simulink model "controller"  (R2025a)
settings: Solver=VariableStepAuto  StartTime=0.0  StopTime=20  RelTol=1e-3
values from neighbouring files (symbols this model uses):
  qd = [0 5.20948749525e-05 0.00020837949981 0.000468853874573 0.000833517999241 0.00130237187381 0.00187541549829 0.00255264887267 0.00333407199696 0.00421968487116 0.00520948749525 0.00630347986926 ... (2700 elements, 450x6)]    [dq.mat]
undefined symbols (not defined in the file or in its folder): D, ddqd, dqd, new_time, Q, rou
(part 2 of 2)

== matlab function controller/robot/MATLAB Function2 ==
  data: q input size=6*1; n_hat output size=6*1; dq input size=6*1
function n_hat = fcn(q, dq)
th = q;
dth = dq;
th1 = th(1); th2 = th(2); th3 = th(3); th4 = th(4); th5 = th(5); th6 = th(6);
dth1 = dth(1); dth2 = dth(2); dth3 = dth(3); dth4 = dth(4); dth5 = dth(5); dth6 = dth(6);
% % ddth1 = ddth(1); ddth2 = ddth(2); ddth3 = ddth(3); ddth4 = ddth(4); ddth5 = ddth(5); ddth6 = ddth(6);

G = [0;
    (1866843*sin(th2 - th3 + th4 + th5))/2000000 - (795688119*sin(th2 - th3))/25000000 - (1866843*sin(th2 - th3 + th4 - th5))/2000000 - (40439763*sin(th2 - th3 + th4))/6250000 - (689642019*sin(th2))/12500000;
     (795688119*sin(th2 - th3))/25000000 - (1866843*sin(th2 - th3 + th4 + th5))/2000000 + (1866843*sin(th2 - th3 + th4 - th5))/2000000 + (40439763*sin(th2 - th3 + th4))/6250000;
     (1866843*sin(th2 - th3 + th4 + th5))/2000000 - (1866843*sin(th2 - th3 + th4 - th5))/2000000 - (40439763*sin(th2 - th3 + th4))/6250000;
     (1866843*sin(th2 - th3 + th4 + th5))/2000000 + (1866843*sin(th2 - th3 + th4 - th5))/2000000;
     0];

C = [(138917031*dth2^2*sin(th2))/250000000 - (5709*dth2^2*sin(th2 - th3 + th4 + th5))/2500000 - (5709*dth3^2*sin(th2 - th3 + th4 + th5))/2500000 - (5709*dth4^2*sin(th2 - th3 + th4 + th5))/2500000 - (173173*dth5^2*sin(th2 - th3 + th4 + th5))/5000000 + (2438609*dth2^2*sin(th2 - th3))/6250000 + (2438609*dth3^2*sin(th2 - th3))/6250000 + (378697*dth2^2*sin(th2 - th5))/10000000 - (378697*dth5^2*sin(th2 - th5))/10000000 + (173173*dth2^2*sin(th2 - th3 + th4 - th5))/5000000 + (2389*dth2^2*sin(th2 - th3 + th4 - 2*th5))/1250000 - (2389*dth2^2*sin(th2 - th3 + th4 + 2*th5))/1250000 + (173173*dth3^2*sin(th2 - th3 + th4 - th5))/5000000 + (2389*dth3^2*sin(th2 - th3 + th4 - 2*th5))/1250000 - (2389*dth3^2*sin(th2 - th3 + th4 + 2*th5))/1250000 + (173173*dth4^2*sin(th2 - th3 + th4 - th5))/5000000 + (2389*dth4^2*sin(th2 - th3 + th4 - 2*th5))/1250000 - (2389*dth4^2*sin(th2 - th3 + th4 + 2*th5))/1250000 + (5709*dth5^2*sin(th2 - th3 + th4 - th5))/2500000 + (3998631*dth2^2*sin(th2 - th3 + th4))/31250000 + (17127*dth2^2*sin(th2 - th3 + th5))/500000 - (17127*dth2^2*sin(th3 - th2 + th5))/500000 + (3998631*dth3^2*sin(th2 - th3 + th4))/31250000 + (17127*dth3^2*sin(th2 - th3 + th5))/500000 - (17127*dth3^2*sin(th3 - th2 + th5))/500000 + (3998631*dth4^2*sin(th2 - th3 + th4))/31250000 - (17127*dth5^2*sin(th2 - th3 + th5))/500000 + (17127*dth5^2*sin(th3 - th2 + th5))/500000 + (378697*dth2^2*sin(th2 + th5))/10000000 - (378697*dth5^2*sin(th2 + th5))/10000000 - (161408701*dth1*dth3*sin(th3))/125000000 - (371007*dth1*dth4*sin(th4))/1562500 - (184591*dth1*dth5*sin(th5))/2500000 + (8203377*dth1*dth2*sin(2*th2 - th3 + th4))/15625000 + (371007*dth1*dth2*sin(2*th2 - 2*th3 + th4))/781250 - (8203377*dth1*dth3*sin(2*th2 - th3 + th4))/31250000 - (371007*dth1*dth3*sin(2*th2 - 2*th3 + th4))/781250 + (8203377*dth1*dth4*sin(2*th2 - th3 + th4))/31250000 + (371007*dth1*dth4*sin(2*th2 - 2*th3 + th4))/1562500 + (5709*dth2*dth3*sin(th2 - th3 + th4 + th5))/1250000 - (5709*dth2*dth4*sin(th2 - th3 + th4 + th5))/1250000 - (184591*dth2*dth5*sin(th2 - th3 + th4 + th5))/5000000 + (5709*dth3*dth4*sin(th2 - th3 + th4 + th5))/1250000 + (dth2*dth6*sin(th2 - th3 + th4 + th5))/20000 + (184591*dth3*dth5*sin(th2 - th3 + th4 + th5))/5000000 - (dth3*dth6*sin(th2 - th3 + th4 + th5))/20000 - (184591*dth4*dth5*sin(th2 - th3 + th4 + th5))/5000000 + (dth4*dth6*sin(th2 - th3 + th4 + th5))/20000 + (dth5*dth6*sin(th2 - th3 + th4 + th5))/20000 - (2438609*dth2*dth3*sin(th2 - th3))/3125000 - (8203377*dth1*dth3*sin(th3 - th4))/31250000 + (8203377*dth1*dth4*sin(th3 - th4))/31250000 - (17127*dth1*dth4*sin(th4 - th5))/500000 + (17127*dth1*dth5*sin(th4 - th5))/500000 + (32351*dth1*dth2*sin(2*th2 - 2*th3 + 2*th4 - th5))/1000000 + (2389*dth1*dth2*sin(2*th2 - 2*th3 + 2*th4 - 2*th5))/1250000 + (2389*dth1*dth2*sin(2*th2 - 2*th3 + 2*th4 + 2*th5))/1250000 - (32351*dth1*dth3*sin(2*th2 - 2*th3 + 2*th4 - th5))/1000000 - (2389*dth1*dth3*sin(2*th2 - 2*th3 + 2*th4 - 2*th5))/1250000 - (2389*dth1*dth3*sin(2*th2 - 2*th3 + 2*th4 + 2*th5))/1250000 + (32351*dth1*dth4*sin(2*th2 - 2*th3 + 2*th4 - th5))/1000000 + (2389*dth1*dth4*sin(2*th2 - 2*th3 + 2*th4 - 2*th5))/1250000 + (2389*dth1*dth4*sin(2*th2 - 2*th3 + 2*th4 + 2*th5))/1250000 - (32351*dth1*dth5*sin(2*th2 - 2*th3 + 2*th4 - th5))/2000000 - (2389*dth1*dth5*sin(2*th2 - 2*th3 + 2*th4 - 2*th5))/1250000 + (2389*dth1*dth5*sin(2*th2 - 2*th3 + 2*th4 + 2*th5))/1250000 + (212507419*dth1*dth2*sin(2*th2))/125000000 - (2389*dth1*dth5*sin(2*th5))/625000 + (526847*dth1*dth2*sin(2*th2 - 2*th3 + 2*th4))/6250000 - (526847*dth1*dth3*sin(2*th2 - 2*th3 + 2*th4))/6250000 + (526847*dth1*dth4*sin(2*th2 - 2*th3 + 2*th4))/6250000 - (378697*dth1*dth2*sin(2*th2 - th3 + th4 + th5))/5000000 - (17127*dth1*dth2*sin(2*th2 - 2*th3 + th4 + th5))/250000 + (378697*dth1*dth3*sin(2*th2 - th3 + th4 + th5))/10000000 - (173173*dth2*dth3*sin(th2 - th3 + th4 - th5))/2500000 + (17127*dth1*dth3*sin(2*th2 - 2*th3 + th4 + th5))/250000 - (378697*dth1*dth4*sin(2*th2 - th3 + th4 + th5))/10000000 - (2389*dth2*dth3*sin(th2 - th3 + th4 - 2*th5))/625000 + (2389*dth2*dth3*sin(th2 - th3 + th4 + 2*th5))/625000 + (173173*dth2*dth4*sin(th2 - th3 + th4 - th5))/2500000 - (17127*dth1*dth4*sin(2*th2 - 2*th3 + th4 + th5))/500000 - (378697*dth1*dth5*sin(2*th2 - th3 + th4 + th5))/10000000 + (2389*dth2*dth4*sin(th2 - th3 + th4 - 2*th5))/625000 - (2389*dth2*dth4*sin(th2 - th3 + th4 + 2*th5))/625000 - (184591*dth2*dth5*sin(th2 - th3 + th4 - th5))/5000000 - (173173*dth3*dth4*sin(th2 - th3 + th4 - th5))/2500000 - (17127*dth1*dth5*sin(2*th2 - 2*th3 + th4 + th5))/500000 - (2389*dth2*dth5*sin(th2 - th3 + th4 - 2*th5))/625000 - (2389*dth2*dth5*sin(th2 - th3 + th4 + 2*th5))/625000 - (dth2*dth6*sin(th2 - th3 + th4 - th5))/20000 - (2389*dth3*dth4*sin(th2 - th3 + th4 - 2*th5))/625000 + (2389*dth3*dth4*sin(th2 - th3 + th4 + 2*th5))/625000 + (184591*dth3*dth5*sin(th2 - th3 + th4 - th5))/5000000 + (2389*dth3*dth5*sin(th2 - th3 + th4 - 2*th5))/625000 + (2389*dth3*dth5*sin(th2 - th3 + th4 + 2*th5))/625000 + (dth3*dth6*sin(th2 - th3 + th4 - th5))/20000 - (184591*dth4*dth5*sin(th2 - th3 + th4 - th5))/5000000 - (2389*dth4*dth5*sin(th2 - th3 + th4 - 2*th5))/625000 - (2389*dth4*dth5*sin(th2 - th3 + th4 + 2*th5))/625000 - (dth4*dth6*sin(th2 - th3 + th4 - th5))/20000 + (dth5*dth6*sin(th2 - th3 + th4 - th5))/20000 + (161408701*dth1*dth2*sin(2*th2 - th3))/62500000 + (509639*dth1*dth2*sin(2*th2 - 2*th3))/625000 - (161408701*dth1*dth3*sin(2*th2 - th3))/125000000 - (509639*dth1*dth3*sin(2*th2 - 2*th3))/625000 - (3998631*dth2*dth3*sin(th2 - th3 + th4))/15625000 - (17127*dth2*dth3*sin(th2 - th3 + th5))/250000 + (17127*dth2*dth3*sin(th3 - th2 + th5))/250000 + (3998631*dth2*dth4*sin(th2 - th3 + th4))/15625000 - (378697*dth1*dth3*sin(th3 - th4 + th5))/10000000 - (378697*dth1*dth3*sin(th4 - th3 + th5))/10000000 - (13431*dth2*dth5*sin(th2 - th3 + th4))/1250000 - (3998631*dth3*dth4*sin(th2 - th3 + th4))/15625000 + (378697*dth1*dth4*sin(th3 - th4 + th5))/10000000 + (378697*dth1*dth4*sin(th4 - th3 + th5))/10000000 + (13431*dth3*dth5*sin(th2 - th3 + th4))/1250000 - (378697*dth1*dth5*sin(th3 - th4 + th5))/10000000 + (378697*dth1*dth5*sin(th4 - th3 + th5))/10000000 - (13431*dth4*dth5*sin(th2 - th3 + th4))/1250000 + (17127*dth1*dth4*sin(th4 + th5))/500000 + (17127*dth1*dth5*sin(th4 + th5))/500000 + (378697*dth1*dth2*sin(2*th2 - th3 + th4 - th5))/5000000 + (17127*dth1*dth2*sin(2*th2 - 2*th3 + th4 - th5))/250000 - (378697*dth1*dth3*sin(2*th2 - th3 + th4 - th5))/10000000 - (32351*dth1*dth2*sin(2*th2 - 2*th3 + 2*th4 + th5))/1000000 - (17127*dth1*dth3*sin(2*th2 - 2*th3 + th4 - th5))/250000 + (378697*dth1*dth4*sin(2*th2 - th3 + th4 - th5))/10000000 + (32351*dth1*dth3*sin(2*th2 - 2*th3 + 2*th4 + th5))/1000000 + (17127*dth1*dth4*sin(2*th2 - 2*th3 + th4 - th5))/500000 - (378697*dth1*dth5*sin(2*th2 - th3 + th4 - th5))/10000000 - (32351*dth1*dth4*sin(2*th2 - 2*th3 + 2*th4 + th5))/1000000 - (17127*dth1*dth5*sin(2*th2 - 2*th3 + th4 - th5))/500000 - (32351*dth1*dth5*sin(2*th2 - 2*th3 + 2*th4 + th5))/2000000;
(161408701*dth3^2*sin(th3))/125000000 - (371007*dth4^2*sin(th4))/1562500 + (32351*dth5^2*sin(th5))/1000000 - (8203377*dth1^2*sin(2*th2 - th3 + th4))/31250000 - (371007*dth1^2*sin(2*th2 - 2*th3 + th4))/1562500 + (8203377*dth3^2*sin(th3 - th4))/31250000 + (8203377*dth4^2*sin(th3 - th4))/31250000 - (17127*dth4^2*sin(th4 - th5))/500000 - (17127*dth5^2*sin(th4 - th5))/500000 - (32351*dth1^2*sin(2*th2 - 2*th3 + 2*th4 - th5))/2000000 - (2389*dth1^2*sin(2*th2 - 2*th3 + 2*th4 - 2*th5))/2500000 - (2389*dth1^2*sin(2*th2 - 2*th3 + 2*th4 + 2*th5))/2500000 - (212507419*dth1^2*sin(2*th2))/250000000 - (526847*dth1^2*sin(2*th2 - 2*th3 + 2*th4))/12500000 + (378697*dth1^2*sin(2*th2 - th3 + th4 + th5))/10000000 + (17127*dth1^2*sin(2*th2 - 2*th3 + th4 + th5))/500000 - (161408701*dth1^2*sin(2*th2 - th3))/125000000 - (509639*dth1^2*sin(2*th2 - 2*th3))/1250000 + (378697*dth3^2*sin(th3 - th4 + th5))/10000000 + (378697*dth3^2*sin(th4 - th3 + th5))/10000000 + (378697*dth4^2*sin(th3 - th4 + th5))/10000000 + (378697*dth4^2*sin(th4 - th3 + th5))/10000000 + (378697*dth5^2*sin(th3 - th4 + th5))/10000000 + (378697*dth5^2*sin(th4 - th3 + th5))/10000000 + (17127*dth4^2*sin(th4 + th5))/500000 + (17127*dth5^2*sin(th4 + th5))/500000 - (378697*dth1^2*sin(2*th2 - th3 + th4 - th5))/10000000 - (17127*dth1^2*sin(2*th2 - 2*th3 + th4 - th5))/500000 + (32351*dth1^2*sin(2*th2 - 2*th3 + 2*th4 + th5))/2000000 - (161408701*dth2*dth3*sin(th3))/62500000 - (371007*dth2*dth4*sin(th4))/781250 + (371007*dth3*dth4*sin(th4))/781250 - (dth5*dth6*sin(th5))/10000 + (32351*dth1*dth5*sin(th2 - th3 + th4 + th5))/1000000 - (dth1*dth6*sin(th2 - th3 + th4 + th5))/20000 - (8203377*dth2*dth3*sin(th3 - th4))/15625000 - (378697*dth1*dth5*sin(th2 - th5))/5000000 + (8203377*dth2*dth4*sin(th3 - th4))/15625000 - (8203377*dth3*dth4*sin(th3 - th4))/15625000 - (17127*dth2*dth4*sin(th4 - th5))/250000 + (17127*dth2*dth5*sin(th4 - th5))/250000 + (17127*dth3*dth4*sin(th4 - th5))/250000 - (17127*dth3*dth5*sin(th4 - th5))/250000 + (17127*dth4*dth5*sin(th4 - th5))/250000 + (2389*dth2*dth5*sin(2*th5))/312500 - (2389*dth3*dth5*sin(2*th5))/312500 + (2389*dth4*dth5*sin(2*th5))/312500 - (32351*dth1*dth5*sin(th2 - th3 + th4 - th5))/1000000 - (2389*dth1*dth5*sin(th2 - th3 + th4 - 2*th5))/625000 - (2389*dth1*dth5*sin(th2 - th3 + th4 + 2*th5))/625000 + (dth1*dth6*sin(th2 - th3 + th4 - th5))/20000 + (13431*dth1*dth5*sin(th2 - th3 + th4))/1250000 + (17127*dth1*dth5*sin(th2 - th3 + th5))/250000 + (17127*dth1*dth5*sin(th3 - th2 + th5))/250000 - (378697*dth2*dth3*sin(th3 - th4 + th5))/5000000 - (378697*dth2*dth3*sin(th4 - th3 + th5))/5000000 + (378697*dth2*dth4*sin(th3 - th4 + th5))/5000000 + (378697*dth2*dth4*sin(th4 - th3 + th5))/5000000 - (378697*dth2*dth5*sin(th3 - th4 + th5))/5000000 + (378697*dth2*dth5*sin(th4 - th3 + th5))/5000000 - (378697*dth3*dth4*sin(th3 - th4 + th5))/5000000 - (378697*dth3*dth4*sin(th4 - th3 + th5))/5000000 + (378697*dth3*dth5*sin(th3 - th4 + th5))/5000000 - (378697*dth3*dth5*sin(th4 - th3 + th5))/5000000 - (378697*dth4*dth5*sin(th3 - th4 + th5))/5000000 + (378697*dth4*dth5*sin(th4 - th3 + th5))/5000000 + (378697*dth1*dth5*sin(th2 + th5))/5000000 + (17127*dth2*dth4*sin(th4 + th5))/250000 + (17127*dth2*dth5*sin(th4 + th5))/250000 - (17127*dth3*dth4*sin(th4 + th5))/250000 - (17127*dth3*dth5*sin(th4 + th5))/250000 + (17127*dth4*dth5*sin(th4 + th5))/250000;
(161408701*dth1^2*sin(th3))/250000000 + (161408701*dth2^2*sin(th3))/125000000 + (371007*dth4^2*sin(th4))/1562500 - (32351*dth5^2*sin(th5))/1000000 + (8203377*dth1^2*sin(2*th2 - th3 + th4))/62500000 + (371007*dth1^2*sin(2*th2 - 2*th3 + th4))/1562500 + (8203377*dth1^2*sin(th3 - th4))/62500000 + (8203377*dth2^2*sin(th3 - th4))/31250000 + (17127*dth4^2*sin(th4 - th5))/500000 + (17127*dth5^2*sin(th4 - th5))/500000 + (32351*dth1^2*sin(2*th2 - 2*th3 + 2*th4 - th5))/2000000 + (2389*dth1^2*sin(2*th2 - 2*th3 + 2*th4 - 2*th5))/2500000 + (2389*dth1^2*sin(2*th2 - 2*th3 + 2*th4 + 2*th5))/2500000 + (526847*dth1^2*sin(2*th2 - 2*th3 + 2*th4))/12500000 - (378697*dth1^2*sin(2*th2 - th3 + th4 + th5))/20000000 - (17127*dth1^2*sin(2*th2 - 2*th3 + th4 + th5))/500000 + (161408701*dth1^2*sin(2*th2 - th3))/250000000 + (509639*dth1^2*sin(2*th2 - 2*th3))/1250000 + (378697*dth1^2*sin(th3 - th4 + th5))/20000000 + (378697*dth1^2*sin(th4 - th3 + th5))/20000000 + (378697*dth2^2*sin(th3 - th4 + th5))/10000000 + (378697*dth2^2*sin(th4 - th3 + th5))/10000000 - (17127*dth4^2*sin(th4 + th5))/500000 - (17127*dth5^2*sin(th4 + th5))/500000 + (378697*dth1^2*sin(2*th2 - th3 + th4 - th5))/20000000 + (17127*dth1^2*sin(2*th2 - 2*th3 + th4 - th5))/500000 - (32351*dth1^2*sin(2*th2 - 2*th3 + 2*th4 + th5))/2000000 + (371007*dth2*dth4*sin(th4))/781250 - (371007*dth3*dth4*sin(th4))/781250 + (dth5*dth6*sin(th5))/10000 - (32351*dth1*dth5*sin(th2 - th3 + th4 + th5))/1000000 + (dth1*dth6*sin(th2 - th3 + th4 + th5))/20000 + (17127*dth2*dth4*sin(th4 - th5))/250000 - (17127*dth2*dth5*sin(th4 - th5))/250000 - (17127*dth3*dth4*sin(th4 - th5))/250000 + (17127*dth3*dth5*sin(th4 - th5))/250000 - (17127*dth4*dth5*sin(th4 - th5))/250000 - (2389*dth2*dth5*sin(2*th5))/312500 + (2389*dth3*dth5*sin(2*th5))/312500 - (2389*dth4*dth5*sin(2*th5))/312500 + (32351*dth1*dth5*sin(th2 - th3 + th4 - th5))/1000000 + (2389*dth1*dth5*sin(th2 - th3 + th4 - 2*th5))/625000 + (2389*dth1*dth5*sin(th2 - th3 + th4 + 2*th5))/625000 - (dth1*dth6*sin(th2 - th3 + th4 - th5))/20000 - (13431*dth1*dth5*sin(th2 - th3 + th4))/1250000 - (17127*dth1*dth5*sin(th2 - th3 + th5))/250000 - (17127*dth1*dth5*sin(th3 - th2 + th5))/250000 - (17127*dth2*dth4*sin(th4 + th5))/250000 - (17127*dth2*dth5*sin(th4 + th5))/250000 + (17127*dth3*dth4*sin(th4 + th5))/250000 + (17127*dth3*dth5*sin(th4 + th5))/250000 - (17127*dth4*dth5*sin(th4 + th5))/250000;
(371007*dth1^2*sin(th4))/3125000 + (371007*dth2^2*sin(th4))/1562500 + (371007*dth3^2*sin(th4))/1562500 + (32351*dth5^2*sin(th5))/1000000 - (8203377*dth1^2*sin(2*th2 - th3 + th4))/62500000 - (371007*dth1^2*sin(2*th2 - 2*th3 + th4))/3125000 - (8203377*dth1^2*sin(th3 - th4))/62500000 - (8203377*dth2^2*sin(th3 - th4))/31250000 + (17127*dth1^2*sin(th4 - th5))/1000000 + (17127*dth2^2*sin(th4 - th5))/500000 + (17127*dth3^2*sin(th4 - th5))/500000 - (32351*dth1^2*sin(2*th2 - 2*th3 + 2*th4 - th5))/2000000 - (2389*dth1^2*sin(2*th2 - 2*th3 + 2*th4 - 2*th5))/2500000 - (2389*dth1^2*sin(2*th2 - 2*th3 + 2*th4 + 2*th5))/2500000 - (526847*dth1^2*sin(2*th2 - 2*th3 + 2*th4))/12500000 + (378697*dth1^2*sin(2*th2 - th3 + th4 + th5))/20000000 + (17127*dth1^2*sin(2*th2 - 2*th3 + th4 + th5))/1000000 - (378697*dth1^2*sin(th3 - th4 + th5))/20000000 - (378697*dth1^2*sin(th4 - th3 + th5))/20000000 - (378697*dth2^2*sin(th3 - th4 + th5))/10000000 - (378697*dth2^2*sin(th4 - th3 + th5))/10000000 - (17127*dth1^2*sin(th4 + th5))/1000000 - (17127*dth2^2*sin(th4 + th5))/500000 - (17127*dth3^2*sin(th4 + th5))/500000 - (378697*dth1^2*sin(2*th2 - th3 + th4 - th5))/20000000 - (17127*dth1^2*sin(2*th2 - 2*th3 + th4 - th5))/1000000 + (32351*dth1^2*sin(2*th2 - 2*th3 + 2*th4 + th5))/2000000 - (371007*dth2*dth3*sin(th4))/781250 - (dth5*dth6*sin(th5))/10000 + (32351*dth1*dth5*sin(th2 - th3 + th4 + th5))/1000000 - (dth1*dth6*sin(th2 - th3 + th4 + th5))/20000 - (17127*dth2*dth3*sin(th4 - th5))/250000 + (2389*dth2*dth5*sin(2*th5))/312500 - (2389*dth3*dth5*sin(2*th5))/312500 + (2389*dth4*dth5*sin(2*th5))/312500 - (32351*dth1*dth5*sin(th2 - th3 + th4 - th5))/1000000 - (2389*dth1*dth5*sin(th2 - th3 + th4 - 2*th5))/625000 - (2389*dth1*dth5*sin(th2 - th3 + th4 + 2*th5))/625000 + (dth1*dth6*sin(th2 - th3 + th4 - th5))/20000 + (13431*dth1*dth5*sin(th2 - th3 + th4))/1250000 + (17127*dth2*dth3*sin(th4 + th5))/250000;
(184591*dth1^2*sin(th5))/5000000 - (17127*dth1^2*sin(th4 - th5))/1000000 - (17127*dth2^2*sin(th4 - th5))/500000 - (17127*dth3^2*sin(th4 - th5))/500000 + (32351*dth1^2*sin(2*th2 - 2*th3 + 2*th4 - th5))/4000000 + (2389*dth1^2*sin(2*th2 - 2*th3 + 2*th4 - 2*th5))/2500000 - (2389*dth1^2*sin(2*th2 - 2*th3 + 2*th4 + 2*th5))/2500000 + (2389*dth1^2*sin(2*th5))/1250000 - (2389*dth2^2*sin(2*th5))/625000 - (2389*dth3^2*sin(2*th5))/625000 - (2389*dth4^2*sin(2*th5))/625000 + (378697*dth1^2*sin(2*th2 - th3 + th4 + th5))/20000000 + (17127*dth1^2*sin(2*th2 - 2*th3 + th4 + th5))/1000000 + (378697*dth1^2*sin(th3 - th4 + th5))/20000000 - (378697*dth1^2*sin(th4 - th3 + th5))/20000000 + (378697*dth2^2*sin(th3 - th4 + th5))/10000000 - (378697*dth2^2*sin(th4 - th3 + th5))/10000000 - (17127*dth1^2*sin(th4 + th5))/1000000 - (17127*dth2^2*sin(th4 + th5))/500000 - (17127*dth3^2*sin(th4 + th5))/500000 + (378697*dth1^2*sin(2*th2 - th3 + th4 - th5))/20000000 + (17127*dth1^2*sin(2*th2 - 2*th3 + th4 - th5))/1000000 + (32351*dth1^2*sin(2*th2 - 2*th3 + 2*th4 + th5))/4000000 + (dth2*dth6*sin(th5))/10000 - (dth3*dth6*sin(th5))/10000 + (dth4*dth6*sin(th5))/10000 - (32351*dth1*dth2*sin(th2 - th3 + th4 + th5))/1000000 + (32351*dth1*dth3*sin(th2 - th3 + th4 + th5))/1000000 - (32351*dth1*dth4*sin(th2 - th3 + th4 + th5))/1000000 - (dth1*dth6*sin(th2 - th3 + th4 + th5))/20000 + (378697*dth1*dth2*sin(th2 - th5))/5000000 + (17127*dth2*dth3*sin(th4 - th5))/250000 + (2389*dth2*dth3*sin(2*th5))/312500 - (2389*dth2*dth4*sin(2*th5))/312500 + (2389*dth3*dth4*sin(2*th5))/312500 + (32351*dth1*dth2*sin(th2 - th3 + th4 - th5))/1000000 + (2389*dth1*dth2*sin(th2 - th3 + th4 - 2*th5))/625000 + (2389*dth1*dth2*sin(th2 - th3 + th4 + 2*th5))/625000 - (32351*dth1*dth3*sin(th2 - th3 + th4 - th5))/1000000 - (2389*dth1*dth3*sin(th2 - th3 + th4 - 2*th5))/625000 - (2389*dth1*dth3*sin(th2 - th3 + th4 + 2*th5))/625000 + (32351*dth1*dth4*sin(th2 - th3 + th4 - th5))/1000000 + (2389*dth1*dth4*sin(th2 - th3 + th4 - 2*th5))/625000 + (2389*dth1*dth4*sin(th2 - th3 + th4 + 2*th5))/625000 - (dth1*dth6*sin(th2 - th3 + th4 - th5))/20000 - (13431*dth1*dth2*sin(th2 - th3 + th4))/1250000 - (17127*dth1*dth2*sin(th2 - th3 + th5))/250000 - (17127*dth1*dth2*sin(th3 - th2 + th5))/250000 + (13431*dth1*dth3*sin(th2 - th3 + th4))/1250000 + (17127*dth1*dth3*sin(th2 - th3 + th5))/250000 + (17127*dth1*dth3*sin(th3 - th2 + th5))/250000 - (13431*dth1*dth4*sin(th2 - th3 + th4))/1250000 - (378697*dth1*dth2*sin(th2 + th5))/5000000 + (17127*dth2*dth3*sin(th4 + th5))/250000;
0];

n_hat = zeros(6,1);

n_hat = C+G;

== matlab function controller/Robustness/MATLAB Function ==
  data: qh input; y output; dqh input; D input; Q input; rou input
function y = w(qh,dqh,D,Q,rou)
z=D.'*Q*[qh;dqh];
% y=rou*sign(z);
% y=rou*z/max(norm(z),7.88*1e-5);
y=rou*tanh(z);
% y=zeros(6,1);
% a=1;
% for i=1:length(z)
%     if z(i)<-1
%         z(i)=-a;
%     elseif z(i)<1
%         z(i)=a*z(i);
%     else
%         z(i)=a;
%     end
% end
% y=rou*z;

== matlab function controller/qd1/MATLAB Function ==
  data: new_time input; y output size=6*1; qd input; t input
function y = fcn(new_time, qd, t)

y = interp1(new_time,qd,t,"linear")';

== matlab function controller/qd1/MATLAB Function1 ==
  data: new_time input; y output size=6*1; dqd input; t input
function y = fcn(new_time, dqd, t)

y = interp1(new_time(1:length(new_time)-1),dqd,t,"linear")';

== matlab function controller/qd1/MATLAB Function2 ==
  data: new_time input; y output size=6*1; ddqd input; t input
function y = fcn(new_time, ddqd, t)

y = interp1(new_time(1:length(new_time)-2),ddqd,t,"linear")';
